simulink model "gyro_synthetic_data"  (R2014a)
settings: Solver=FixedStepDiscrete  StartTime=0.0  StopTime=t_sim  FixedStep=t_step  RelTol=1e-3
undefined symbols (not defined in the file or in its folder): omega_B
libraries: lib_gyro_fusion x4
settings Model: Creator=kirill  LastModifiedBy=kirill

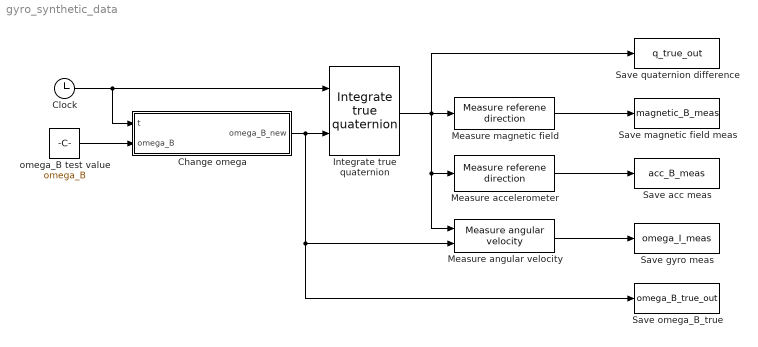
== system gyro_synthetic_data ==
  Change omega : MATLAB Function  TreatAsAtomicUnit=on
  Clock : Clock
  Integrate true quaternion : lib_gyro_fusion/Integrate true quaternion  q_BI_init=q_init
  Measure accelerometer : lib_gyro_fusion/Measure referene direction  ref_direction=gravity_I  measurement_noise_power=acc_noise_power  measurement_sample_rate=t_step  source_seeds=acc_seeds  R_direction=R_acc
  Measure angular velocity : lib_gyro_fusion/Measure angular velocity
  Measure magnetic field : lib_gyro_fusion/Measure referene direction  ref_direction=ref_B_I  measurement_noise_power=magnetometer_noise_power  measurement_sample_rate=t_step  source_seeds=magnetometer_seeds  R_direction=R_magnetometer
  Save acc meas : ToWorkspace  VariableName=acc_B_meas  SaveFormat=Timeseries  SampleTime=-1
  Save gyro meas : ToWorkspace  VariableName=omega_I_meas  SaveFormat=Timeseries  SampleTime=-1
  Save magnetic field meas : ToWorkspace  VariableName=magnetic_B_meas  SaveFormat=Timeseries  SampleTime=-1
  Save omega_B_true : ToWorkspace  VariableName=omega_B_true_out  SaveFormat=Timeseries  SampleTime=-1
  Save quaternion difference : ToWorkspace  VariableName=q_true_out  SaveFormat=Timeseries  SampleTime=-1
  omega_B test value : Constant  Value=omega_B
  wires:
  Clock/1 -> Change omega/1(t), Integrate true quaternion/1
  Integrate true quaternion/1 -> Measure angular velocity/1, Measure accelerometer/1, Measure magnetic field/1, Save quaternion difference/1
  Change omega/1(omega_B_new) -> Save omega_B_true/1, Measure angular velocity/2, Integrate true quaternion/2
  omega_B test value/1 -> Change omega/2(omega_B)
  Measure magnetic field/1 -> Save magnetic field meas/1
  Measure accelerometer/1 -> Save acc meas/1
  Measure angular velocity/1 -> Save gyro meas/1

== matlab function gyro_synthetic_data/Change omega ==
  data: t input; omega_B input; omega_B_new output
function omega_B_new = change_omega(t, omega_B)
%#codegen
a = [cos(2 * pi * t / 120); cos(2 * pi * t / 20.5); cos(2 * pi * t / 81.5)];
omega_B_new = a.* omega_B;
